simulink model "ex2"  (R2023b)
settings: Solver=VariableStepAuto  StartTime=0.0  StopTime=10.0  RelTol=1e-3
settings Model: Creator=Andrei  LastModifiedBy=Andrei

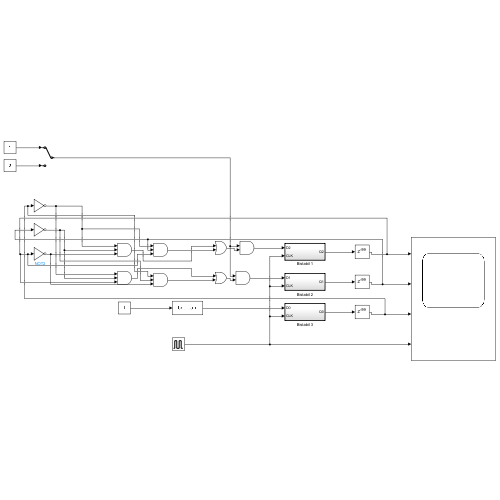
[thumbnail: Simulink's stored preview of the top-level diagram]
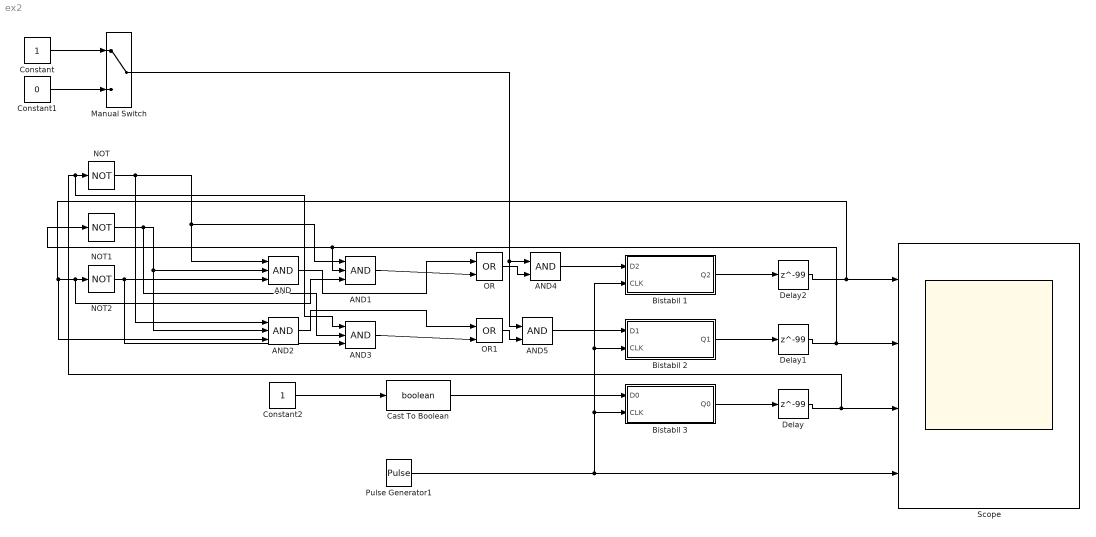
== system ex2 ==
  AND{,1..3} (4 alike) : Logic  Inputs=3  IconShape=distinctive  AllPortsSameDT=off  OutDataTypeStr=boolean
  AND4 : Logic  IconShape=distinctive  AllPortsSameDT=off  OutDataTypeStr=boolean
  AND5 : Logic  IconShape=distinctive  AllPortsSameDT=off  OutDataTypeStr=boolean
  Bistabil 1 : Subsystem  TreatAsAtomicUnit=on
  Bistabil 2 : Subsystem  TreatAsAtomicUnit=on
  Bistabil 3 : Subsystem  TreatAsAtomicUnit=on
  Cast To Boolean : DataTypeConversion  OutDataTypeStr=boolean  SaturateOnIntegerOverflow=off  RndMeth=Floor
  Constant : Constant
  Constant1 : Constant  Value=0
  Constant2 : Constant
  Delay : Delay  DelayLength=99
  Delay1 : Delay  DelayLength=99
  Delay2 : Delay  DelayLength=99
  Manual Switch : ManualSwitch
  NOT : Logic  Operator=NOT  IconShape=distinctive  AllPortsSameDT=off  OutDataTypeStr=boolean
  NOT1 : Logic  Operator=NOT  IconShape=distinctive  AllPortsSameDT=off  OutDataTypeStr=boolean
  NOT2 : Logic  Operator=NOT  IconShape=distinctive  AllPortsSameDT=off  OutDataTypeStr=boolean
  OR : Logic  Operator=OR  IconShape=distinctive  AllPortsSameDT=off  OutDataTypeStr=boolean
  OR1 : Logic  Operator=OR  IconShape=distinctive  AllPortsSameDT=off  OutDataTypeStr=boolean
  Pulse Generator1 : DiscretePulseGenerator  PulseType=Time based  PulseWidth=5
  Scope : Scope  NumInputPorts=4
  wires:
  Constant2/1 -> Cast To Boolean/1
  Constant1/1 -> Manual Switch/2
  Pulse Generator1/1 -> Scope/4, Bistabil 1/2(CLK), Bistabil 2/2(CLK), Bistabil 3/2(CLK)
  Bistabil 2/1(Q1) -> Delay1/1
  Constant/1 -> Manual Switch/1
  Delay2/1 -> AND2/3, AND1/3, NOT2/1, Scope/1
  Delay1/1 -> NOT1/1, AND1/2, Scope/2
  Bistabil 3/1(Q0) -> Delay/1
  Bistabil 1/1(Q2) -> Delay2/1
  Cast To Boolean/1 -> Bistabil 3/1(D0)
  AND3/1 -> OR1/2
  AND2/1 -> OR1/1
  AND1/1 -> OR/2
  AND/1 -> OR/1
  NOT/1 -> AND2/1, AND1/1, AND/1
  NOT1/1 -> AND3/2, AND2/2, AND/2
  NOT2/1 -> AND3/3, AND/3
  Delay/1 -> AND3/1, NOT/1, Scope/3
  AND4/1 -> Bistabil 1/1(D2)
  OR/1 -> AND4/2
  Manual Switch/1 -> AND5/1, AND4/1
  AND5/1 -> Bistabil 2/1(D1)
  OR1/1 -> AND5/2

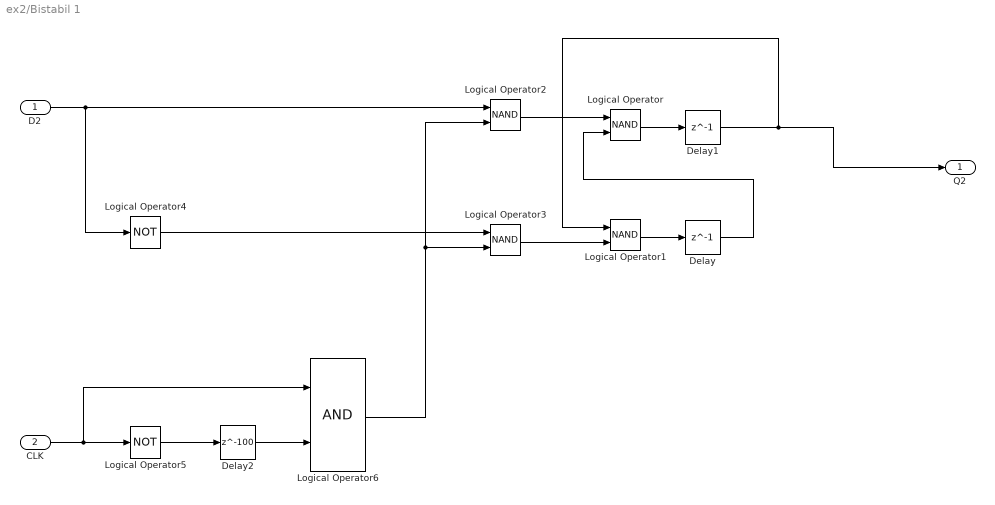
== system ex2/Bistabil 1 ==
  D2 : Inport
  CLK : Inport  Port=2
  Delay : Delay  DelayLength=1  InitialCondition=0
  Delay1 : Delay  DelayLength=1  InitialCondition=0
  Delay2 : Delay  DelayLength=100  InitialCondition=0
  Logical Operator{,1..3} (4 alike) : Logic  Operator=NAND  AllPortsSameDT=off  OutDataTypeStr=boolean
  Logical Operator4 : Logic  Operator=NOT  AllPortsSameDT=off  OutDataTypeStr=boolean
  Logical Operator5 : Logic  Operator=NOT  AllPortsSameDT=off  OutDataTypeStr=boolean
  Logical Operator6 : Logic  AllPortsSameDT=off  OutDataTypeStr=boolean
  Q2 : Outport
  wires:
  D2/1 -> Logical Operator4/1, Logical Operator2/1
  CLK/1 -> Logical Operator6/1, Logical Operator5/1
  Delay1/1 -> Logical Operator1/1, Q2/1
  Logical Operator5/1 -> Delay2/1
  Delay2/1 -> Logical Operator6/2
  Logical Operator4/1 -> Logical Operator3/1
  Logical Operator6/1 -> Logical Operator3/2, Logical Operator2/2
  Logical Operator3/1 -> Logical Operator1/2
  Logical Operator2/1 -> Logical Operator/1
  Logical Operator/1 -> Delay1/1
  Logical Operator1/1 -> Delay/1
  Delay/1 -> Logical Operator/2

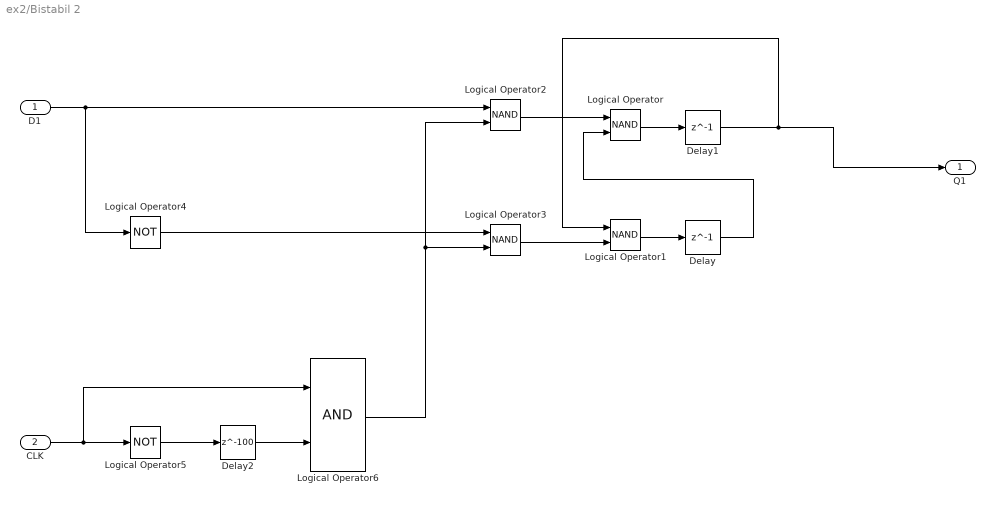
== system ex2/Bistabil 2 ==
  D1 : Inport
  CLK : Inport  Port=2
  Delay : Delay  DelayLength=1  InitialCondition=0
  Delay1 : Delay  DelayLength=1  InitialCondition=0
  Delay2 : Delay  DelayLength=100  InitialCondition=0
  Logical Operator{,1..3} (4 alike) : Logic  Operator=NAND  AllPortsSameDT=off  OutDataTypeStr=boolean
  Logical Operator4 : Logic  Operator=NOT  AllPortsSameDT=off  OutDataTypeStr=boolean
  Logical Operator5 : Logic  Operator=NOT  AllPortsSameDT=off  OutDataTypeStr=boolean
  Logical Operator6 : Logic  AllPortsSameDT=off  OutDataTypeStr=boolean
  Q1 : Outport
  wires:
  D1/1 -> Logical Operator4/1, Logical Operator2/1
  CLK/1 -> Logical Operator6/1, Logical Operator5/1
  Delay1/1 -> Logical Operator1/1, Q1/1
  Logical Operator5/1 -> Delay2/1
  Delay2/1 -> Logical Operator6/2
  Logical Operator4/1 -> Logical Operator3/1
  Logical Operator6/1 -> Logical Operator3/2, Logical Operator2/2
  Logical Operator3/1 -> Logical Operator1/2
  Logical Operator2/1 -> Logical Operator/1
  Logical Operator/1 -> Delay1/1
  Logical Operator1/1 -> Delay/1
  Delay/1 -> Logical Operator/2

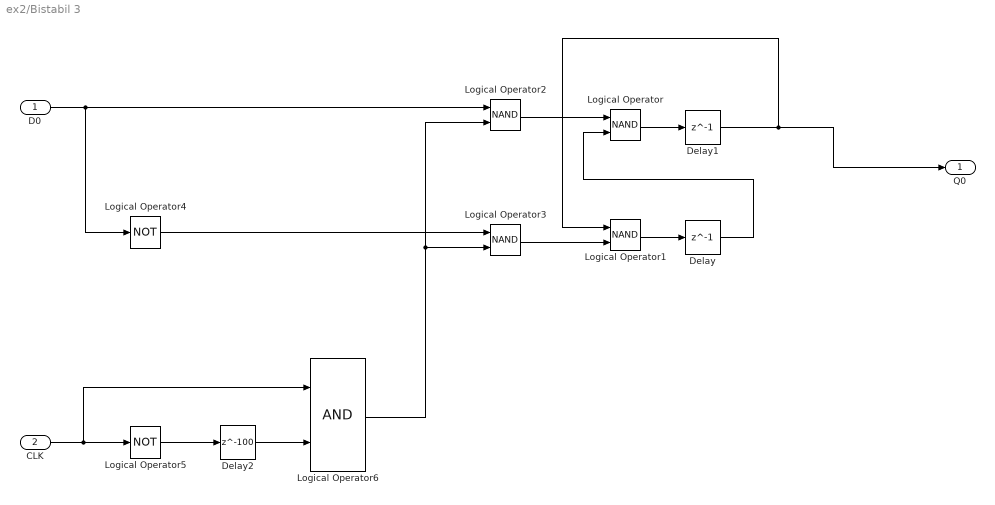
== system ex2/Bistabil 3 ==
  D0 : Inport
  CLK : Inport  Port=2
  Delay : Delay  DelayLength=1  InitialCondition=0
  Delay1 : Delay  DelayLength=1  InitialCondition=0
  Delay2 : Delay  DelayLength=100  InitialCondition=0
  Logical Operator{,1..3} (4 alike) : Logic  Operator=NAND  AllPortsSameDT=off  OutDataTypeStr=boolean
  Logical Operator4 : Logic  Operator=NOT  AllPortsSameDT=off  OutDataTypeStr=boolean
  Logical Operator5 : Logic  Operator=NOT  AllPortsSameDT=off  OutDataTypeStr=boolean
  Logical Operator6 : Logic  AllPortsSameDT=off  OutDataTypeStr=boolean
  Q0 : Outport
  wires:
  D0/1 -> Logical Operator4/1, Logical Operator2/1
  CLK/1 -> Logical Operator6/1, Logical Operator5/1
  Delay1/1 -> Logical Operator1/1, Q0/1
  Logical Operator5/1 -> Delay2/1
  Delay2/1 -> Logical Operator6/2
  Logical Operator4/1 -> Logical Operator3/1
  Logical Operator6/1 -> Logical Operator3/2, Logical Operator2/2
  Logical Operator3/1 -> Logical Operator1/2
  Logical Operator2/1 -> Logical Operator/1
  Logical Operator/1 -> Delay1/1
  Logical Operator1/1 -> Delay/1
  Delay/1 -> Logical Operator/2
